simulink model "mlep_fenix_direct_hf_ctrl"  (R2020a)
settings: Solver=VariableStepAuto  StartTime=0.0  StopTime=sim_time  RelTol=1e-3
InitFcn:
  | mlep_fenix_direct_hf_ctrl_init;
values from neighbouring files (symbols this model uses):
  k_i = 0.2    [mlep_fenix_direct_hf_ctrl_init.m]
  k_p = 200    [mlep_fenix_direct_hf_ctrl_init.m]
  max_heat_power = 3500    [mlep_fenix_direct_hf_ctrl_init.m]
undefined symbols (not defined in the file or in its folder): main_seq, max_temp, min_temp, PRNS, seed_1, seed_2, temp_dc, temp_noise_std, Ts_ep, Ts_rand_temp
libraries: simulink x13, mlepLibrary x1
settings Model: Creator=Tomáš  LastModifiedBy=baumetom
settings DataIOCC: ReturnWorkspaceOutputs=off
settings DebuggingCC: PregeneratedLibrarySubsystemCodeDiagnostic=none  ArithmeticOperatorsInVariantConditions=warning
settings SFSimCC: SimUseLocalCustomCode=off  CustomCodeUndefinedFunction=UseInterfaceOnly
settings RTWCC: RTWUseLocalCustomCode=off

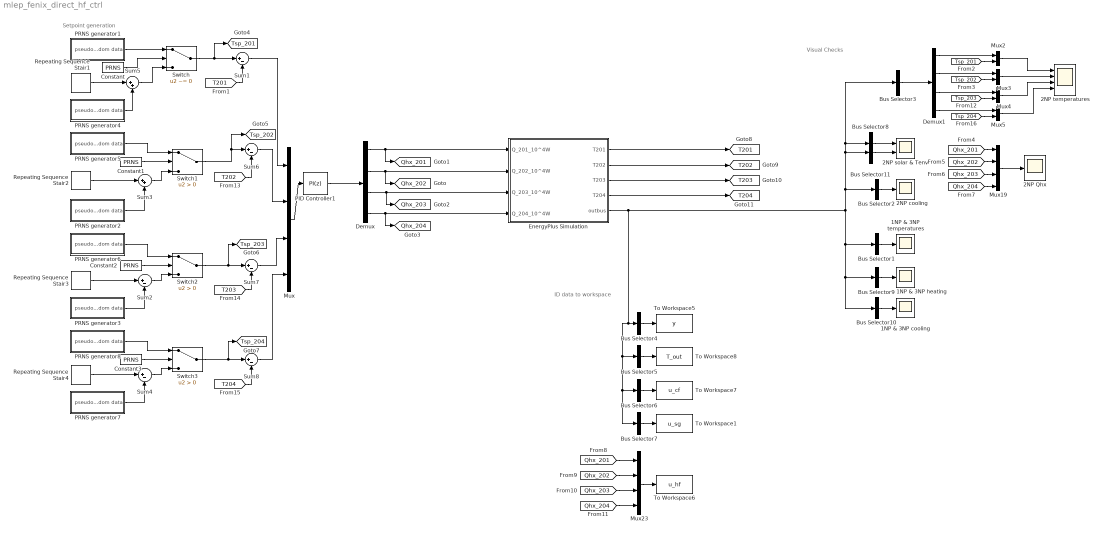
== system mlep_fenix_direct_hf_ctrl ==
  note: Setpoint generation
  note: ID data to workspace
  note: Visual Checks
  1NP & 3NP cooling : Scope
  1NP & 3NP heating : Scope
  1NP & 3NP temperatures : Scope
  "2NP Qhx " : Scope
  2NP cooling : Scope
  2NP solar & Tenv : Scope  NumInputPorts=2
  2NP temperatures : Scope  NumInputPorts=4
  Bus Selector1 : BusSelector  OutputSignals=EP_1NP_1NPX101__Zone_Mean_Air_Temperature,EP_1NP_1NPXSchodiste__Zone_Mean_Air_Temperature,EP_1NP_1NPX103__Zone_Mean_Air_Temperature,EP_3NP_3NPX301XStrojovna__Zone_Mean_Air_Temperature,EP_3NP_3NPXSchodiste__Zone_Mean_Air_Temperature,EP_3NP_3NPX303__Zone_Mean_Air_Temperature  OutputAsBus=on
  Bus Selector10 : BusSelector  OutputSignals=EP_1NP_1NPX101__Zone_Air_System_Sensible_Cooling_Rate,EP_1NP_1NPXSchodiste__Zone_Air_System_Sensible_Cooling_Rate,EP_1NP_1NPX103__Zone_Air_System_Sensible_Cooling_Rate,EP_3NP_3NPX301XStrojovna__Zone_Air_System_Sensible_Cooling_Rate,EP_3NP_3NPXSchodiste__Zone_Air_System_Sensible_Cooling_Rate,EP_3NP_3NPX303__Zone_Air_System_Sensible_Cooling_Rate  OutputAsBus=on
  Bus Selector11 : BusSelector  OutputSignals=EP_Environment__Site_Outdoor_Air_Drybulb_Temperature  OutputAsBus=on
  Bus Selector2 : BusSelector  OutputSignals=EP_2NP_2NPXSchodiste__Zone_Air_System_Sensible_Cooling_Rate,EP_2NP_2NPX202__Zone_Air_System_Sensible_Cooling_Rate,EP_2NP_2NPX203__Zone_Air_System_Sensible_Cooling_Rate,EP_2NP_2NPX204__Zone_Air_System_Sensible_Cooling_Rate  OutputAsBus=on
  Bus Selector3 : BusSelector  OutputSignals=EP_2NP_2NPXSchodiste__Zone_Mean_Air_Temperature,EP_2NP_2NPX202__Zone_Mean_Air_Temperature,EP_2NP_2NPX203__Zone_Mean_Air_Temperature,EP_2NP_2NPX204__Zone_Mean_Air_Temperature  OutputAsBus=on
  Bus Selector4 : BusSelector  OutputSignals=EP_2NP_2NPXSchodiste__Zone_Mean_Air_Temperature,EP_2NP_2NPX202__Zone_Mean_Air_Temperature,EP_2NP_2NPX203__Zone_Mean_Air_Temperature,EP_2NP_2NPX204__Zone_Mean_Air_Temperature  OutputAsBus=on
  Bus Selector5 : BusSelector  OutputSignals=EP_Environment__Site_Outdoor_Air_Drybulb_Temperature  OutputAsBus=on
  Bus Selector6 : BusSelector  OutputSignals=EP_2NP_2NPXSchodiste__Zone_Air_System_Sensible_Cooling_Rate,EP_2NP_2NPX202__Zone_Air_System_Sensible_Cooling_Rate,EP_2NP_2NPX203__Zone_Air_System_Sensible_Cooling_Rate,EP_2NP_2NPX204__Zone_Air_System_Sensible_Cooling_Rate  OutputAsBus=on
  Bus Selector7 : BusSelector  OutputSignals=EP_2NP_2NPXSchodiste__Zone_Windows_Total_Transmitted_Solar_Radiation_Rate,EP_2NP_2NPX202__Zone_Windows_Total_Transmitted_Solar_Radiation_Rate,EP_2NP_2NPX203__Zone_Windows_Total_Transmitted_Solar_Radiation_Rate,EP_2NP_2NPX204__Zone_Windows_Total_Transmitted_Solar_Radiation_Rate  OutputAsBus=on
  Bus Selector8 : BusSelector  OutputSignals=EP_2NP_2NPXSchodiste__Zone_Windows_Total_Transmitted_Solar_Radiation_Rate,EP_2NP_2NPX202__Zone_Windows_Total_Transmitted_Solar_Radiation_Rate,EP_2NP_2NPX203__Zone_Windows_Total_Transmitted_Solar_Radiation_Rate,EP_2NP_2NPX204__Zone_Windows_Total_Transmitted_Solar_Radiation_Rate  OutputAsBus=on
  Bus Selector9 : BusSelector  OutputSignals=EP_1NP_1NPX101__Zone_Air_System_Sensible_Heating_Rate,EP_1NP_1NPX101__Zone_People_Sensible_Heating_Rate,EP_1NP_1NPXSchodiste__Zone_Air_System_Sensible_Heating_Rate,EP_1NP_1NPX103__Zone_Air_System_Sensible_Heating_Rate,EP_1NP_1NPX103__Zone_People_Sensible_Heating_Rate,EP_3NP_3NPX301XStrojovna__Zone_Air_System_Sensible_Heating_Rate,EP_3NP_3NPXSchodiste__Zone_Air_System_Sensible_Heating_Rate,EP_3NP_3NPX303__Zone_Air_System_Sensible_Heating_Rate,EP_3NP_3NPX303__Zone_People_Sensible_Heating_Rate  OutputAsBus=on
  Constant{,1..3} (4 alike) : Constant  Value=PRNS
  Demux : Demux
  Demux1 : Demux
  EnergyPlus Simulation : Subsystem  Priority=2
      mask Display: image('Fenix.PNG')
  Mux : Mux
  Mux19 : Mux
  Mux{2..5} (4 alike) : Mux  Inputs=2
  Mux23 : Mux
  PID Controller1 : simulink/Continuous/PID Controller  Controller=PI  Form=Parallel  TimeDomain=Discrete-time  UseExternalTs=off  SampleTime=-1  IntegratorMethod=Forward Euler  FilterMethod=Forward Euler  ControllerParametersSource=internal  P=k_p  I=k_i  D=0  UseFilter=on  N=100  TunerSelectOption=Transfer Function Based (PID Tuner App)  InitialConditionSource=internal  InitialConditionForIntegrator=0  InitialConditionForFilter=0  DifferentiatorICPrevScaledInput=0  ExternalReset=none  TrackingMode=off  Kt=1  LimitOutput=on  UpperSaturationLimit=max_heat_power(1)  LowerSaturationLimit=0  LinearizeAsGain=on  AntiWindupMode=clamping  Kb=1  POutMin=[]  POutMax=[]  IOutMin=[]  IOutMax=[]  DOutMin=[]  DOutMax=[]  NOutMin=[]  NOutMax=[]  SumOutMin=[]  SumOutMax=[]  SaturationOutMin=[]  SaturationOutMax=[]  PParamMin=[]  PParamMax=[]  IParamMin=[]  IParamMax=[]  DParamMin=[]  DParamMax=[]  NParamMin=[]  NParamMax=[]  KbParamMin=[]  KbParamMax=[]  KtParamMin=[]  KtParamMax=[]  KbOutMin=[]  KbOutMax=[]  KtOutMin=[]  KtOutMax=[]  IntegratorOutMin=[]  IntegratorOutMax=[]  FilterOutMin=[]  FilterOutMax=[]  SumI1OutMin=[]  SumI1OutMax=[]  SumI2OutMin=[]  SumI2OutMax=[]  SumI3OutMin=[]  SumI3OutMax=[]  SumI4OutMin=[]  SumI4OutMax=[]  SumDOutMin=[]  SumDOutMax=[]  DifferentiatorOutMin=[]  DifferentiatorOutMax=[]  FilterDiffOutCoefMin=[]  FilterDiffOutCoefMax=[]  ReciprocalOutMin=[]  ReciprocalOutMax=[]  SumDenOutMin=[]  SumDenOutMax=[]  SumNumOutMin=[]  SumNumOutMax=[]  DivideOutMin=[]  DivideOutMax=[]  UdiffTsProdOutMin=[]  UdiffTsProdOutMax=[]  NTsProdOutMin=[]  NTsProdOutMax=[]  UintegralTsProdOutMin=[]  UintegralTsProdOutMax=[]  UngainTsProdOutMin=[]  UngainTsProdOutMax=[]  IntegratorContinuousStateAttributes=''  IntegratorStateMustResolveToSignalObject=off  IntegratorRTWStateStorageClass=Auto  FilterContinuousStateAttributes=''  FilterStateMustResolveToSignalObject=off  FilterRTWStateStorageClass=Auto  ParallelPVariant=InternalParameters  IdealPVariant=Disabled  IVariant=InternalParameters  DVariant=Disabled  IntegratorVariant=Discrete  SatVariant=Enabled  AWVariant=DiscClampingParallel  PCopyVariant=Disabled  TRVariant=Disabled  FdbkBlocksVariant=Forward  IdealPFdbkVariant=Disabled  SatFdbkVariant=Disabled  DerivativeFilterVariant=Disabled  NVariant=Disabled  NCopyVariant=Disabled_SignalSpec  FilterICVariant=Disabled  IntegratorICVariant=InternalICs  ExternalResetVariant=Disabled  TRSumVariant=Passthrough  SumFdbkVariant=Disabled  SumVariant=Sum_PI  TsampFilterVariant=InternalTs  TsampNgainVariant=Passthrough  TsampIntegralVariant=Passthrough
  PRNS generator1 : Subsystem  mask{temp_dc=temp_dc(1), temp_std=temp_noise_std(1), temp_min=min_temp(1), temp_max=max_temp(1), Ts_rand=Ts_rand_temp(1), Ts=Ts_ep, seed=seed_1(1)}
      mask prompts: temp_dc "Mean temperature [°C]"; temp_std "Temperature deviation [°C]"; temp_min "Minimal temperature [°C]"; temp_max "Maximal temperature [°C]"; Ts_rand "Sequence period [s]"; Ts "Sample time [s]"; seed "Seed [-]"
      mask DialogControl DescGroupVar Prompt: PseudoRandom Number Sequence Generator
  PRNS generator2 : Subsystem  mask{temp_dc=temp_dc(2), temp_std=temp_noise_std(2), temp_min=min_temp(2), temp_max=max_temp(2), Ts_rand=Ts_rand_temp(2), Ts=Ts_ep, seed=seed_2(2)}
      mask prompts: temp_dc "Mean temperature [°C]"; temp_std "Temperature deviation [°C]"; temp_min "Minimal temperature [°C]"; temp_max "Maximal temperature [°C]"; Ts_rand "Sequence period [s]"; Ts "Sample time [s]"; seed "Seed [-]"
      mask DialogControl DescGroupVar Prompt: PseudoRandom Number Sequence Generator
  PRNS generator3 : Subsystem  mask{temp_dc=temp_dc(2), temp_std=temp_noise_std(2), temp_min=min_temp(2), temp_max=max_temp(2), Ts_rand=Ts_rand_temp(2), Ts=Ts_ep, seed=seed_2(3)}
      mask prompts: temp_dc "Mean temperature [°C]"; temp_std "Temperature deviation [°C]"; temp_min "Minimal temperature [°C]"; temp_max "Maximal temperature [°C]"; Ts_rand "Sequence period [s]"; Ts "Sample time [s]"; seed "Seed [-]"
      mask DialogControl DescGroupVar Prompt: PseudoRandom Number Sequence Generator
  PRNS generator4 : Subsystem  mask{temp_dc=temp_dc(2), temp_std=temp_noise_std(2), temp_min=min_temp(2), temp_max=max_temp(2), Ts_rand=Ts_rand_temp(2), Ts=Ts_ep, seed=seed_2(1)}
      mask prompts: temp_dc "Mean temperature [°C]"; temp_std "Temperature deviation [°C]"; temp_min "Minimal temperature [°C]"; temp_max "Maximal temperature [°C]"; Ts_rand "Sequence period [s]"; Ts "Sample time [s]"; seed "Seed [-]"
      mask DialogControl DescGroupVar Prompt: PseudoRandom Number Sequence Generator
  PRNS generator5 : Subsystem  mask{temp_dc=temp_dc(1), temp_std=temp_noise_std(1), temp_min=min_temp(1), temp_max=max_temp(1), Ts_rand=Ts_rand_temp(1), Ts=Ts_ep, seed=seed_1(2)}
      mask prompts: temp_dc "Mean temperature [°C]"; temp_std "Temperature deviation [°C]"; temp_min "Minimal temperature [°C]"; temp_max "Maximal temperature [°C]"; Ts_rand "Sequence period [s]"; Ts "Sample time [s]"; seed "Seed [-]"
      mask DialogControl DescGroupVar Prompt: PseudoRandom Number Sequence Generator
  PRNS generator6 : Subsystem  mask{temp_dc=temp_dc(1), temp_std=temp_noise_std(1), temp_min=min_temp(1), temp_max=max_temp(1), Ts_rand=Ts_rand_temp(1), Ts=Ts_ep, seed=seed_1(3)}
      mask prompts: temp_dc "Mean temperature [°C]"; temp_std "Temperature deviation [°C]"; temp_min "Minimal temperature [°C]"; temp_max "Maximal temperature [°C]"; Ts_rand "Sequence period [s]"; Ts "Sample time [s]"; seed "Seed [-]"
      mask DialogControl DescGroupVar Prompt: PseudoRandom Number Sequence Generator
  PRNS generator7 : Subsystem  mask{temp_dc=temp_dc(2), temp_std=temp_noise_std(2), temp_min=min_temp(2), temp_max=max_temp(2), Ts_rand=Ts_rand_temp(2), Ts=Ts_ep, seed=seed_2(4)}
      mask prompts: temp_dc "Mean temperature [°C]"; temp_std "Temperature deviation [°C]"; temp_min "Minimal temperature [°C]"; temp_max "Maximal temperature [°C]"; Ts_rand "Sequence period [s]"; Ts "Sample time [s]"; seed "Seed [-]"
      mask DialogControl DescGroupVar Prompt: PseudoRandom Number Sequence Generator
  PRNS generator8 : Subsystem  mask{temp_dc=temp_dc(1), temp_std=temp_noise_std(1), temp_min=min_temp(1), temp_max=max_temp(1), Ts_rand=Ts_rand_temp(1), Ts=Ts_ep, seed=seed_1(4)}
      mask prompts: temp_dc "Mean temperature [°C]"; temp_std "Temperature deviation [°C]"; temp_min "Minimal temperature [°C]"; temp_max "Maximal temperature [°C]"; Ts_rand "Sequence period [s]"; Ts "Sample time [s]"; seed "Seed [-]"
      mask DialogControl DescGroupVar Prompt: PseudoRandom Number Sequence Generator
  Repeating Sequence Stair1 : simulink/Sources/Repeating Sequence Stair  OutValues=main_seq(1,:)  tsamp=Ts_rand_temp(1)  OutMin=[]  OutMax=[]  OutDataTypeStr=double  OutputDataTypeScalingMode=double  OutDataType=fixdt(0,8)  ConRadixGroup=Best Precision: Vector-wise  OutScaling=2^-12
  Repeating Sequence Stair2 : simulink/Sources/Repeating Sequence Stair  OutValues=main_seq(2,:)  tsamp=Ts_rand_temp(1)  OutMin=[]  OutMax=[]  OutDataTypeStr=double  OutputDataTypeScalingMode=double  OutDataType=fixdt(0,8)  ConRadixGroup=Best Precision: Vector-wise  OutScaling=2^-12
  Repeating Sequence Stair3 : simulink/Sources/Repeating Sequence Stair  OutValues=main_seq(3,:)  tsamp=Ts_rand_temp(1)  OutMin=[]  OutMax=[]  OutDataTypeStr=double  OutputDataTypeScalingMode=double  OutDataType=fixdt(0,8)  ConRadixGroup=Best Precision: Vector-wise  OutScaling=2^-12
  Repeating Sequence Stair4 : simulink/Sources/Repeating Sequence Stair  OutValues=main_seq(4,:)  tsamp=Ts_rand_temp(1)  OutMin=[]  OutMax=[]  OutDataTypeStr=double  OutputDataTypeScalingMode=double  OutDataType=fixdt(0,8)  ConRadixGroup=Best Precision: Vector-wise  OutScaling=2^-12
  Sum{1..2,4,6..8} (6 alike) : Sum  Inputs=|+-
  Sum3 : Sum  Inputs=|++
  Sum5 : Sum  Inputs=|++
  Switch : Switch  Criteria=u2 ~= 0
  Switch1 : Switch  Criteria=u2 > Threshold
  Switch2 : Switch  Criteria=u2 > Threshold
  Switch3 : Switch  Criteria=u2 > Threshold
  To Workspace1 : ToWorkspace  VariableName=u_sg  SampleTime=-1
  To Workspace5 : ToWorkspace  VariableName=y  SampleTime=-1
  To Workspace6 : ToWorkspace  VariableName=u_hf  SampleTime=-1
  To Workspace7 : ToWorkspace  VariableName=u_cf  SampleTime=-1
  To Workspace8 : ToWorkspace  VariableName=T_out  SampleTime=-1
      settings: Save2DSignal=2-D array (concatenate along first dimension)
  tag scope: Qhx_201=global, Qhx_202=global, Qhx_203=global, Qhx_204=global, T201=global, T202=global, T203=global, T204=global, Tsp_201=global, Tsp_202=global, Tsp_203=global, Tsp_204=global
  wires:
  Mux19/1 -> "2NP Qhx "/1
  Repeating Sequence Stair2/1 -> Sum3/1
  Repeating Sequence Stair3/1 -> Sum2/1
  Repeating Sequence Stair4/1 -> Sum4/1
  Mux/1 -> PID Controller1/1
  PID Controller1/1 -> Demux/1
  Demux/1 -> [Qhx_201], EnergyPlus Simulation/1(Q_201_10^4W)
  Demux/2 -> [Qhx_202], EnergyPlus Simulation/2(Q_202_10^4W)
  Demux/3 -> [Qhx_203], EnergyPlus Simulation/3(Q_203_10^4W)
  Demux/4 -> [Qhx_204], EnergyPlus Simulation/4(Q_204_10^4W)
  EnergyPlus Simulation/1(T201) -> [T201]
  EnergyPlus Simulation/2(T202) -> [T202]
  EnergyPlus Simulation/3(T203) -> [T203]
  EnergyPlus Simulation/4(T204) -> [T204]
  Bus Selector4/1 -> To Workspace5/1
  Bus Selector5/1 -> To Workspace8/1
  [Qhx_201] -> Mux23/1
  Mux23/1 -> To Workspace6/1
  [Qhx_203] -> Mux23/3
  [Qhx_204] -> Mux23/4
  [Qhx_202] -> Mux23/2
  Bus Selector6/1 -> To Workspace7/1
  Bus Selector7/1 -> To Workspace1/1
  Bus Selector3/1 -> Demux1/1
  Bus Selector8/1 -> 2NP solar & Tenv/1
  Bus Selector2/1 -> 2NP cooling/1
  [Qhx_202] -> Mux19/2
  [Qhx_201] -> Mux19/1
  [Qhx_203] -> Mux19/3
  [Qhx_204] -> Mux19/4
  Bus Selector1/1 -> 1NP & 3NP temperatures/1
  Bus Selector9/1 -> 1NP & 3NP heating/1
  Bus Selector10/1 -> 1NP & 3NP cooling/1
  EnergyPlus Simulation/5(outbus) -> Bus Selector10/1, Bus Selector9/1, Bus Selector1/1, Bus Selector3/1, Bus Selector8/1, Bus Selector11/1, Bus Selector2/1, Bus Selector7/1, Bus Selector6/1, Bus Selector5/1, Bus Selector4/1
  Bus Selector11/1 -> 2NP solar & Tenv/2
  PRNS generator4/1(pseudorandom data) -> Sum5/2
  Repeating Sequence Stair1/1 -> Sum5/1
  Switch/1 -> [Tsp_201], Sum1/1
  [T201] -> Sum1/2
  Switch1/1 -> [Tsp_202], Sum6/1
  [T202] -> Sum6/2
  PRNS generator2/1(pseudorandom data) -> Sum3/2
  Switch2/1 -> [Tsp_203], Sum7/1
  Switch3/1 -> [Tsp_204], Sum8/1
  [T203] -> Sum7/2
  PRNS generator3/1(pseudorandom data) -> Sum2/2
  PRNS generator7/1(pseudorandom data) -> Sum4/2
  [T204] -> Sum8/2
  Sum7/1 -> Mux/3
  Sum8/1 -> Mux/4
  Sum6/1 -> Mux/2
  Sum1/1 -> Mux/1
  [Tsp_201] -> Mux2/2
  [Tsp_202] -> Mux3/2
  [Tsp_203] -> Mux4/2
  [Tsp_204] -> Mux5/2
  Demux1/1 -> Mux2/1
  Demux1/2 -> Mux3/1
  Demux1/3 -> Mux4/1
  Demux1/4 -> Mux5/1
  Mux2/1 -> 2NP temperatures/1
  Mux3/1 -> 2NP temperatures/2
  Mux4/1 -> 2NP temperatures/3
  Mux5/1 -> 2NP temperatures/4
  Sum5/1 -> Switch/3
  PRNS generator1/1(pseudorandom data) -> Switch/1
  Constant/1 -> Switch/2
  Constant1/1 -> Switch1/2
  Sum3/1 -> Switch1/3
  PRNS generator5/1(pseudorandom data) -> Switch1/1
  Sum2/1 -> Switch2/3
  Constant2/1 -> Switch2/2
  PRNS generator6/1(pseudorandom data) -> Switch2/1
  Sum4/1 -> Switch3/3
  Constant3/1 -> Switch3/2
  PRNS generator8/1(pseudorandom data) -> Switch3/1

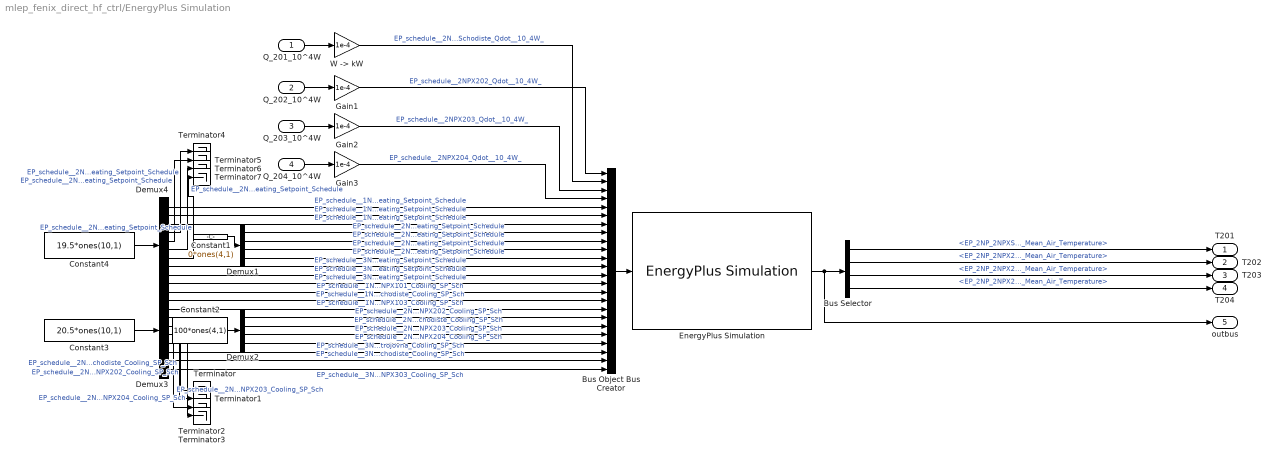
== system mlep_fenix_direct_hf_ctrl/EnergyPlus Simulation ==
  Q_201_10^4W : Inport
  Q_202_10^4W : Inport  Port=2
  Q_203_10^4W : Inport  Port=3
  Q_204_10^4W : Inport  Port=4
  Bus Selector : BusSelector  OutputSignals=EP_2NP_2NPXSchodiste__Zone_Mean_Air_Temperature,EP_2NP_2NPX202__Zone_Mean_Air_Temperature,EP_2NP_2NPX203__Zone_Mean_Air_Temperature,EP_2NP_2NPX204__Zone_Mean_Air_Temperature
  Bus Object Bus Creator : BusCreator  Inputs=24  mask(Bus Object Bus Creator){busType=No Bus objects found.}
      mask prompts: busType "Bus Type"
      mask help:
      | Provides users the cabability to painlessly, instantly customize bus creators of output data type 'Bus:' by selecting the bus object type from a drop down menu dynamically populated by bus objects in the workspace.
      |
      | After pressing the "Apply Selection" button signal lines into the creator are populated and named with the elements in the chosen bus saving the user from having to recall and fill out signal line names.
      |
      | NOTE that when copying a Bus Object Bus Creator from your locked Library the link to the Library is automatically broken. This saves the user from having to Unlock Links To Library (From the Library menu.), Disable Link and finally Break Link (Both from the Model menu.) for every placed instance of the block.
      settings: AttributesFormatString=%<OutDataTypeStr>  CopyFcn=busObjectBusCreator_clbk(gcb,'CopyFcn');
      mask TypeOptions busType: No Bus objects found.
      mask Callback busType: busObjectBusCreator_clbk(gcb,'popup');
      mask DialogControl applyMOCBSelection Prompt: Apply Selection
      mask DialogControl applyMOCBSelection Callback: busObjectBusCreator_clbk(gcb,'button');
  Constant1 : Constant  Value=0*ones(4,1)
  Constant2 : Constant  Value=100*ones(4,1)
  Constant3 : Constant  Value=20.5*ones(10,1)
  Constant4 : Constant  Value=19.5*ones(10,1)
  Demux1 : Demux
  Demux2 : Demux
  Demux3 : Demux  Outputs=10
  Demux4 : Demux  Outputs=10
  EnergyPlus Simulation : mlepLibrary/EnergyPlus Simulation  Priority=1  idfFile=C:\Users\baumetom\OneDrive - České vysoké učení technické v Praze\iq_pump\bitbucket\distributed-grey-box-identification-git\DID_2.0\OOP\models\fenix\Fenix_FDD_ID\fenix_2NP_Heat_off_NO_PEOPLE.idf  epwFile=C:\Users\baumetom\OneDrive - České vysoké učení technické v Praze\iq_pump\bitbucket\distributed-grey-box-identification-git\DID_2.0\OOP\models\fenix\Fenix_FDD_ID\POL_KLODZKO_IMGW.epw  inputBusName=epInbus  outputBusName=epOutbus  useDataDictionary=off  dataDictionaryName=EnergyPlusSimulation.sldd
      settings: SourceProductName=mlep Blocks
  Gain1 : Gain  Gain=1e-4
  Gain2 : Gain  Gain=1e-4
  Gain3 : Gain  Gain=1e-4
  Terminator{,1..7} (8 alike) : Terminator
  "W -> kW" : Gain  Gain=1e-4
  T201 : Outport  VectorParamsAs1DForOutWhenUnconnected=off
  T202 : Outport  Port=2  VectorParamsAs1DForOutWhenUnconnected=off
  T203 : Outport  Port=3  VectorParamsAs1DForOutWhenUnconnected=off
  T204 : Outport  Port=4  VectorParamsAs1DForOutWhenUnconnected=off
  outbus : Outport  Port=5  VectorParamsAs1DForOutWhenUnconnected=off
  wires:
  Demux2/1 -> Bus Object Bus Creator/18  "EP_schedule__2NP_2NPX202_Cooling_SP_Sch"
  Demux4/10 -> Bus Object Bus Creator/14  "EP_schedule__3NP_3NPX303_Heating_Setpoint_Schedule"
  Q_203_10^4W/1 -> Gain2/1
  Demux3/8 -> Bus Object Bus Creator/22  "EP_schedule__3NP_3NPX301XStrojovna_Cooling_SP_Sch"
  Bus Object Bus Creator/1 -> EnergyPlus Simulation/1
  Demux1/1 -> Bus Object Bus Creator/8  "EP_schedule__2NP_2NPX202_Heating_Setpoint_Schedule"
  Demux3/3 -> Bus Object Bus Creator/17  "EP_schedule__1NP_1NPX103_Cooling_SP_Sch"
  Bus Selector/1 -> T201/1  "<EP_2NP_2NPXSchodiste__Zone_Mean_Air_Temperature>"
  Demux4/9 -> Bus Object Bus Creator/13  "EP_schedule__3NP_3NPXSchodiste_Heating_Setpoint_Schedule"
  Gain2/1 -> Bus Object Bus Creator/3  "EP_schedule__2NPX203_Qdot__10_4W_"
  Q_204_10^4W/1 -> Gain3/1
  Q_201_10^4W/1 -> "W -> kW"/1
  Gain1/1 -> Bus Object Bus Creator/1  "EP_schedule__2NPX202_Qdot__10_4W_"
  "W -> kW"/1 -> Bus Object Bus Creator/2  "EP_schedule__2NPXSchodiste_Qdot__10_4W_"
  Demux1/4 -> Bus Object Bus Creator/11  "EP_schedule__2NP_2NPX204_Heating_Setpoint_Schedule"
  Q_202_10^4W/1 -> Gain1/1
  Bus Selector/3 -> T203/1  "<EP_2NP_2NPX203__Zone_Mean_Air_Temperature>"
  Bus Selector/4 -> T204/1  "<EP_2NP_2NPX204__Zone_Mean_Air_Temperature>"
  Demux3/9 -> Bus Object Bus Creator/23  "EP_schedule__3NP_3NPXSchodiste_Cooling_SP_Sch"
  Demux4/1 -> Bus Object Bus Creator/5  "EP_schedule__1NP_1NPX101_Heating_Setpoint_Schedule"
  Demux4/3 -> Bus Object Bus Creator/7  "EP_schedule__1NP_1NPX103_Heating_Setpoint_Schedule"
  Demux4/8 -> Bus Object Bus Creator/12  "EP_schedule__3NP_3NPX301XStrojovna_Heating_Setpoint_Schedule"
  Constant3/1 -> Demux3/1
  Gain3/1 -> Bus Object Bus Creator/4  "EP_schedule__2NPX204_Qdot__10_4W_"
  Demux2/2 -> Bus Object Bus Creator/19  "EP_schedule__2NP_2NPXSchodiste_Cooling_SP_Sch"
  Demux2/3 -> Bus Object Bus Creator/20  "EP_schedule__2NP_2NPX203_Cooling_SP_Sch"
  EnergyPlus Simulation/1 -> outbus/1, Bus Selector/1
  Constant4/1 -> Demux4/1
  Bus Selector/2 -> T202/1  "<EP_2NP_2NPX202__Zone_Mean_Air_Temperature>"
  Demux4/2 -> Bus Object Bus Creator/6  "EP_schedule__1NP_1NPXSchodiste_Heating_Setpoint_Schedule"
  Demux3/10 -> Bus Object Bus Creator/24  "EP_schedule__3NP_3NPX303_Cooling_SP_Sch"
  Demux3/1 -> Bus Object Bus Creator/15  "EP_schedule__1NP_1NPX101_Cooling_SP_Sch"
  Demux1/2 -> Bus Object Bus Creator/9  "EP_schedule__2NP_2NPXSchodiste_Heating_Setpoint_Schedule"
  Demux3/2 -> Bus Object Bus Creator/16  "EP_schedule__1NP_1NPXSchodiste_Cooling_SP_Sch"
  Demux2/4 -> Bus Object Bus Creator/21  "EP_schedule__2NP_2NPX204_Cooling_SP_Sch"
  Demux1/3 -> Bus Object Bus Creator/10  "EP_schedule__2NP_2NPX203_Heating_Setpoint_Schedule"
  Constant1/1 -> Demux1/1
  Constant2/1 -> Demux2/1
  Demux3/4 -> Terminator/1  "EP_schedule__2NP_2NPX202_Cooling_SP_Sch"
  Demux3/5 -> Terminator1/1  "EP_schedule__2NP_2NPXSchodiste_Cooling_SP_Sch"
  Demux3/6 -> Terminator2/1  "EP_schedule__2NP_2NPX203_Cooling_SP_Sch"
  Demux3/7 -> Terminator3/1  "EP_schedule__2NP_2NPX204_Cooling_SP_Sch"
  Demux4/4 -> Terminator4/1  "EP_schedule__2NP_2NPX202_Heating_Setpoint_Schedule"
  Demux4/5 -> Terminator5/1  "EP_schedule__2NP_2NPXSchodiste_Heating_Setpoint_Schedule"
  Demux4/6 -> Terminator6/1  "EP_schedule__2NP_2NPX203_Heating_Setpoint_Schedule"
  Demux4/7 -> Terminator7/1  "EP_schedule__2NP_2NPX204_Heating_Setpoint_Schedule"

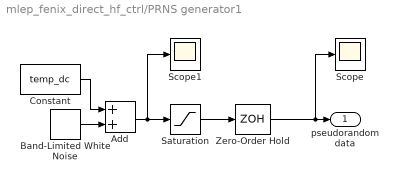
== system mlep_fenix_direct_hf_ctrl/PRNS generator1 ==
  Add : Sum
  Band-Limited White Noise : simulink/Sources/Band-Limited White Noise  Cov=temp_std^2*Ts_rand  Ts=Ts_rand  seed=seed
  Constant : Constant  Value=temp_dc
  Saturation : Saturate  UpperLimit=temp_max  LowerLimit=temp_min
  Scope : Scope
  Scope1 : Scope
  Zero-Order Hold : ZeroOrderHold  SampleTime=Ts
  pseudorandom data : Outport  VectorParamsAs1DForOutWhenUnconnected=off
  wires:
  Saturation/1 -> Zero-Order Hold/1
  Add/1 -> Saturation/1, Scope1/1
  Constant/1 -> Add/1
  Band-Limited White Noise/1 -> Add/2
  Zero-Order Hold/1 -> pseudorandom data/1, Scope/1

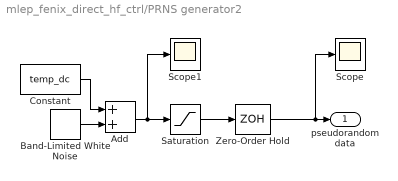
== system mlep_fenix_direct_hf_ctrl/PRNS generator2 ==
  Add : Sum
  Band-Limited White Noise : simulink/Sources/Band-Limited White Noise  Cov=temp_std^2*Ts_rand  Ts=Ts_rand  seed=seed
  Constant : Constant  Value=temp_dc
  Saturation : Saturate  UpperLimit=temp_max  LowerLimit=temp_min
  Scope : Scope
  Scope1 : Scope
  Zero-Order Hold : ZeroOrderHold  SampleTime=Ts
  pseudorandom data : Outport  VectorParamsAs1DForOutWhenUnconnected=off
  wires:
  Saturation/1 -> Zero-Order Hold/1
  Add/1 -> Saturation/1, Scope1/1
  Constant/1 -> Add/1
  Band-Limited White Noise/1 -> Add/2
  Zero-Order Hold/1 -> pseudorandom data/1, Scope/1

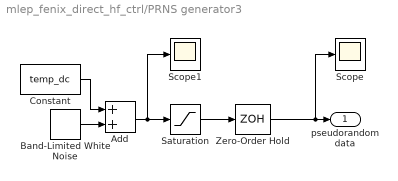
== system mlep_fenix_direct_hf_ctrl/PRNS generator3 ==
  Add : Sum
  Band-Limited White Noise : simulink/Sources/Band-Limited White Noise  Cov=temp_std^2*Ts_rand  Ts=Ts_rand  seed=seed
  Constant : Constant  Value=temp_dc
  Saturation : Saturate  UpperLimit=temp_max  LowerLimit=temp_min
  Scope : Scope
  Scope1 : Scope
  Zero-Order Hold : ZeroOrderHold  SampleTime=Ts
  pseudorandom data : Outport  VectorParamsAs1DForOutWhenUnconnected=off
  wires:
  Zero-Order Hold/1 -> Scope/1, pseudorandom data/1
  Band-Limited White Noise/1 -> Add/2
  Constant/1 -> Add/1
  Add/1 -> Scope1/1, Saturation/1
  Saturation/1 -> Zero-Order Hold/1

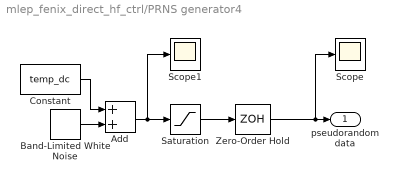
== system mlep_fenix_direct_hf_ctrl/PRNS generator4 ==
  Add : Sum
  Band-Limited White Noise : simulink/Sources/Band-Limited White Noise  Cov=temp_std^2*Ts_rand  Ts=Ts_rand  seed=seed
  Constant : Constant  Value=temp_dc
  Saturation : Saturate  UpperLimit=temp_max  LowerLimit=temp_min
  Scope : Scope
  Scope1 : Scope
  Zero-Order Hold : ZeroOrderHold  SampleTime=Ts
  pseudorandom data : Outport  VectorParamsAs1DForOutWhenUnconnected=off
  wires:
  Zero-Order Hold/1 -> Scope/1, pseudorandom data/1
  Band-Limited White Noise/1 -> Add/2
  Constant/1 -> Add/1
  Add/1 -> Scope1/1, Saturation/1
  Saturation/1 -> Zero-Order Hold/1

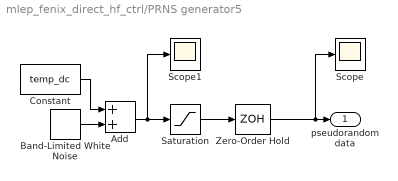
== system mlep_fenix_direct_hf_ctrl/PRNS generator5 ==
  Add : Sum
  Band-Limited White Noise : simulink/Sources/Band-Limited White Noise  Cov=temp_std^2*Ts_rand  Ts=Ts_rand  seed=seed
  Constant : Constant  Value=temp_dc
  Saturation : Saturate  UpperLimit=temp_max  LowerLimit=temp_min
  Scope : Scope
  Scope1 : Scope
  Zero-Order Hold : ZeroOrderHold  SampleTime=Ts
  pseudorandom data : Outport  VectorParamsAs1DForOutWhenUnconnected=off
  wires:
  Zero-Order Hold/1 -> Scope/1, pseudorandom data/1
  Band-Limited White Noise/1 -> Add/2
  Constant/1 -> Add/1
  Add/1 -> Scope1/1, Saturation/1
  Saturation/1 -> Zero-Order Hold/1

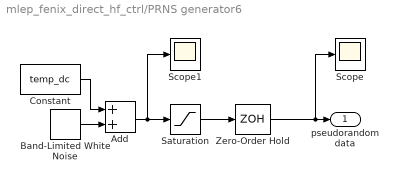
== system mlep_fenix_direct_hf_ctrl/PRNS generator6 ==
  Add : Sum
  Band-Limited White Noise : simulink/Sources/Band-Limited White Noise  Cov=temp_std^2*Ts_rand  Ts=Ts_rand  seed=seed
  Constant : Constant  Value=temp_dc
  Saturation : Saturate  UpperLimit=temp_max  LowerLimit=temp_min
  Scope : Scope
  Scope1 : Scope
  Zero-Order Hold : ZeroOrderHold  SampleTime=Ts
  pseudorandom data : Outport  VectorParamsAs1DForOutWhenUnconnected=off
  wires:
  Saturation/1 -> Zero-Order Hold/1
  Add/1 -> Saturation/1, Scope1/1
  Constant/1 -> Add/1
  Band-Limited White Noise/1 -> Add/2
  Zero-Order Hold/1 -> pseudorandom data/1, Scope/1

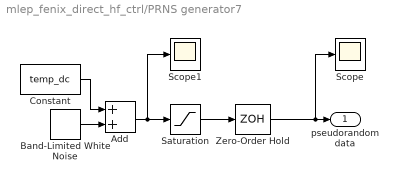
== system mlep_fenix_direct_hf_ctrl/PRNS generator7 ==
  Add : Sum
  Band-Limited White Noise : simulink/Sources/Band-Limited White Noise  Cov=temp_std^2*Ts_rand  Ts=Ts_rand  seed=seed
  Constant : Constant  Value=temp_dc
  Saturation : Saturate  UpperLimit=temp_max  LowerLimit=temp_min
  Scope : Scope
  Scope1 : Scope
  Zero-Order Hold : ZeroOrderHold  SampleTime=Ts
  pseudorandom data : Outport  VectorParamsAs1DForOutWhenUnconnected=off
  wires:
  Saturation/1 -> Zero-Order Hold/1
  Add/1 -> Saturation/1, Scope1/1
  Constant/1 -> Add/1
  Band-Limited White Noise/1 -> Add/2
  Zero-Order Hold/1 -> pseudorandom data/1, Scope/1

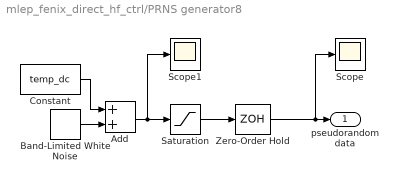
== system mlep_fenix_direct_hf_ctrl/PRNS generator8 ==
  Add : Sum
  Band-Limited White Noise : simulink/Sources/Band-Limited White Noise  Cov=temp_std^2*Ts_rand  Ts=Ts_rand  seed=seed
  Constant : Constant  Value=temp_dc
  Saturation : Saturate  UpperLimit=temp_max  LowerLimit=temp_min
  Scope : Scope
  Scope1 : Scope
  Zero-Order Hold : ZeroOrderHold  SampleTime=Ts
  pseudorandom data : Outport  VectorParamsAs1DForOutWhenUnconnected=off
  wires:
  Zero-Order Hold/1 -> Scope/1, pseudorandom data/1
  Band-Limited White Noise/1 -> Add/2
  Constant/1 -> Add/1
  Add/1 -> Scope1/1, Saturation/1
  Saturation/1 -> Zero-Order Hold/1
